simulink model "ureg"  (Simulink 5.0)
settings: Solver=ode5  StartTime=0.0  StopTime=25  FixedStep=.001  RelTol=1e-3
settings Model: LastModifiedBy=yidier  ExtModeTrigMode=oneshot  ExtModeArmWhenConnect=off  LimitDataPoints=off  BooleanDataType=off

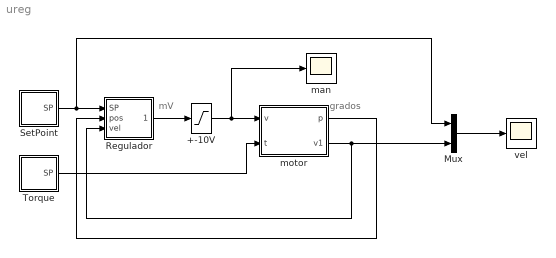
== system ureg ==
  note: mV
  note: grados
  +-10V : Saturate  UpperLimit=10  LowerLimit=-10
  Mux : Mux  Inputs=2
  Regulador : Subsystem
  SetPoint : Subsystem
  Torque : Subsystem
  man : Scope
      settings: TickLabels=on  TimeRange=25  YMin=-1  YMax=1  SaveName=man  DataFormat=Array
  motor : Subsystem
  vel : Scope
      settings: TickLabels=on  TimeRange=5  YMin=-4  YMax=4  SaveName=vel  DataFormat=Array  MaxDataPoints=50000
  wires:
  SetPoint/1(SP) -> Regulador/1(SP), Mux/1
  Regulador/1(man) -> +-10V/1
  +-10V/1 -> man/1, motor/1(v)
  motor/2(v1) -> Regulador/3(vel), Mux/2
  motor/1(p) -> Regulador/2(pos)
  Mux/1 -> vel/1
  Torque/1(SP) -> motor/2(t)

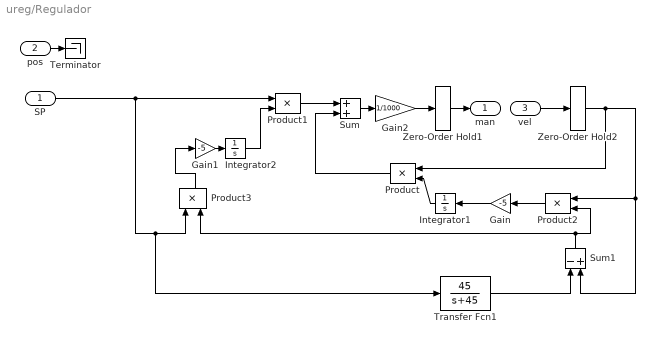
== system ureg/Regulador ==
  SP : Inport
  pos : Inport  Port=2
  vel : Inport  Port=3
  Gain : Gain  Orientation=left  Gain=-5  SaturateOnIntegerOverflow=on
  Gain1 : Gain  Gain=-5  SaturateOnIntegerOverflow=on
  Gain2 : Gain  Gain=1/1000  SaturateOnIntegerOverflow=on
  Integrator1 : Integrator  Orientation=left  InitialCondition=-2
  Integrator2 : Integrator  InitialCondition=2
  Product : Product  Orientation=left  SaturateOnIntegerOverflow=on  InputSameDT=on
  Product1 : Product  SaturateOnIntegerOverflow=on  InputSameDT=on
  Product2 : Product  Orientation=left  SaturateOnIntegerOverflow=on  InputSameDT=on
  Product3 : Product  Orientation=up  SaturateOnIntegerOverflow=on  InputSameDT=on
  Sum : Sum  SaturateOnIntegerOverflow=on  InputSameDT=on
  Sum1 : Sum  Orientation=up  Inputs=-+  SaturateOnIntegerOverflow=on  InputSameDT=on
  Terminator : Terminator
  Transfer Fcn1 : TransferFcn  Numerator=45  Denominator=[1 45]
  Zero-Order Hold1 : ZeroOrderHold  SampleTime=.001
  Zero-Order Hold2 : ZeroOrderHold  SampleTime=.001
  man : Outport
  wires:
  SP/1 -> Product1/1, Transfer Fcn1/1, Product3/1
  pos/1 -> Terminator/1
  Sum/1 -> Gain2/1
  Product1/1 -> Sum/1
  Product/1 -> Sum/2
  Gain/1 -> Integrator1/1
  Product2/1 -> Gain/1
  Gain1/1 -> Integrator2/1
  Sum1/1 -> Product3/2, Product2/2
  Product3/1 -> Gain1/1
  Transfer Fcn1/1 -> Sum1/1
  Integrator2/1 -> Product1/2
  Integrator1/1 -> Product/2
  vel/1 -> Zero-Order Hold2/1
  Gain2/1 -> Zero-Order Hold1/1
  Zero-Order Hold1/1 -> man/1
  Zero-Order Hold2/1 -> Product/1, Product2/1, Sum1/2

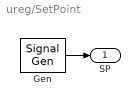
== system ureg/SetPoint ==
  Gen : SignalGenerator  Amplitude=3  Frequency=3  Units=rad/sec
  SP : Outport
  wires:
  Gen/1 -> SP/1

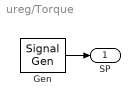
== system ureg/Torque ==
  Gen : SignalGenerator  Amplitude=0  Frequency=3  Units=rad/sec
  SP : Outport
  wires:
  Gen/1 -> SP/1

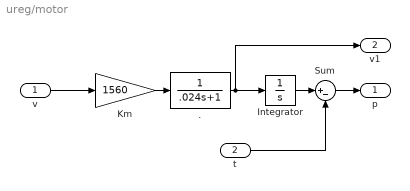
== system ureg/motor ==
  v : Inport
  t : Inport  Port=2
  . : TransferFcn  Numerator=1  Denominator=[.024 1 ]
  Integrator : Integrator
  Km : Gain  Gain=1560  SaturateOnIntegerOverflow=on
  Sum : Sum  Inputs=|+-  SaturateOnIntegerOverflow=on  InputSameDT=on
  p : Outport
  v1 : Outport  Port=2
  wires:
  Km/1 -> ./1
  ./1 -> Integrator/1, v1/1
  v/1 -> Km/1
  Integrator/1 -> Sum/1
  Sum/1 -> p/1
  t/1 -> Sum/2
